simulink model "nigga"  (R2025a)
settings: Solver=VariableStepAuto  StartTime=0.0  StopTime=10.0  RelTol=1e-3
libraries: matlabinput_lib x1
settings Model: Creator=ASUS  LastModifiedBy=ASUS

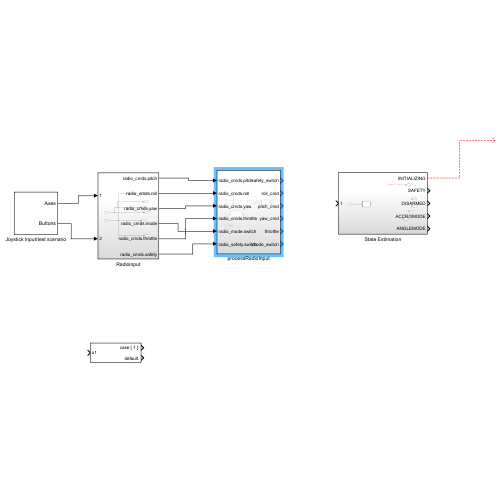
[thumbnail: Simulink's stored preview of the top-level diagram]
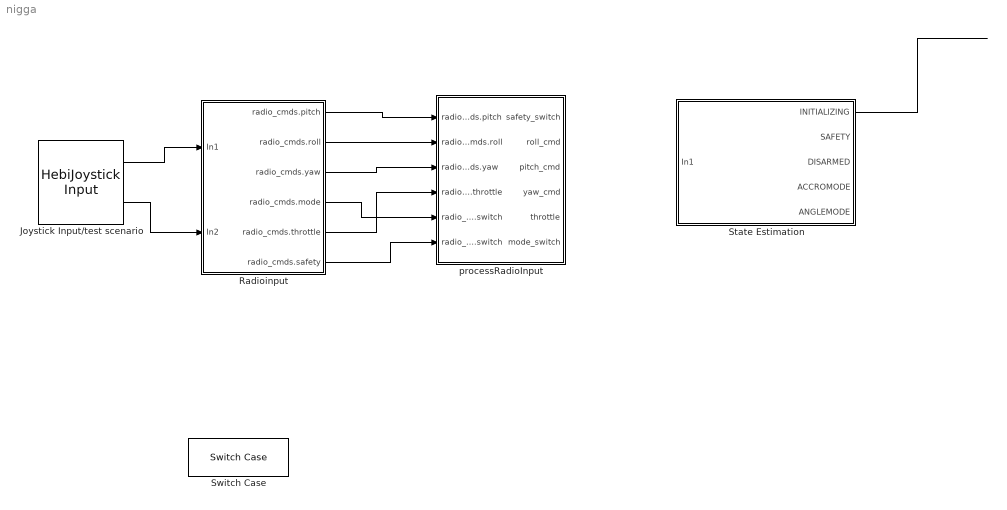
== system nigga ==
  Joystick Input/test scenario : matlabinput_lib/HebiJoystick Input  joyid=1  forcefeed=off
      settings: SourceProductName=MatlabInput
  Radioinput : Subsystem
  State Estimation : Subsystem
  Switch Case : SwitchCase
  processRadioInput : Subsystem
  wires:
  State Estimation/1(INITIALIZING) -> ?
  Joystick Input/test scenario/1 -> Radioinput/1(In1)
  Joystick Input/test scenario/2 -> Radioinput/2(In2)
  Radioinput/1(radio_cmds.pitch) -> processRadioInput/1(radio_cmds.pitch)
  Radioinput/2(radio_cmds.roll) -> processRadioInput/2(radio_cmds.roll)
  Radioinput/3(radio_cmds.yaw) -> processRadioInput/3(radio_cmds.yaw)
  Radioinput/5(radio_cmds.throttle) -> processRadioInput/4(radio_cmds.throttle)
  Radioinput/6(radio_cmds.safety) -> processRadioInput/6(radio_safety.switch)
  Radioinput/4(radio_cmds.mode) -> processRadioInput/5(radio_mode.switch)

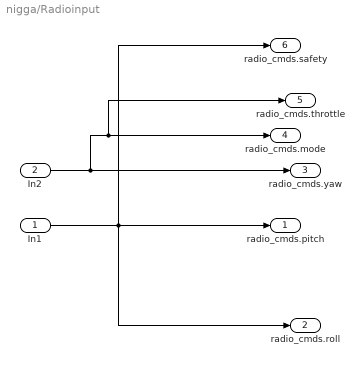
== system nigga/Radioinput ==
  In1 : Inport
  In2 : Inport  Port=2
  radio_cmds.pitch : Outport
  radio_cmds.roll : Outport  Port=2
  radio_cmds.yaw : Outport  Port=3
  radio_cmds.mode : Outport  Port=4
  radio_cmds.throttle : Outport  Port=5
  radio_cmds.safety : Outport  Port=6
  wires:
  In1/1 -> radio_cmds.roll/1, radio_cmds.safety/1, radio_cmds.pitch/1
  In2/1 -> radio_cmds.throttle/1, radio_cmds.mode/1, radio_cmds.yaw/1

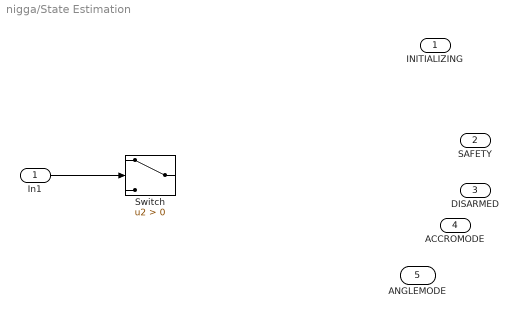
== system nigga/State Estimation ==
  In1 : Inport
  Switch : Switch  Criteria=u2 > Threshold  SaturateOnIntegerOverflow=off  InputSameDT=off
  INITIALIZING : Outport
  SAFETY : Outport  Port=2
  DISARMED : Outport  Port=3
  ACCROMODE : Outport  Port=4
  ANGLEMODE : Outport  Port=5
  wires:
  In1/1 -> Switch/2
  ? -> INITIALIZING/1

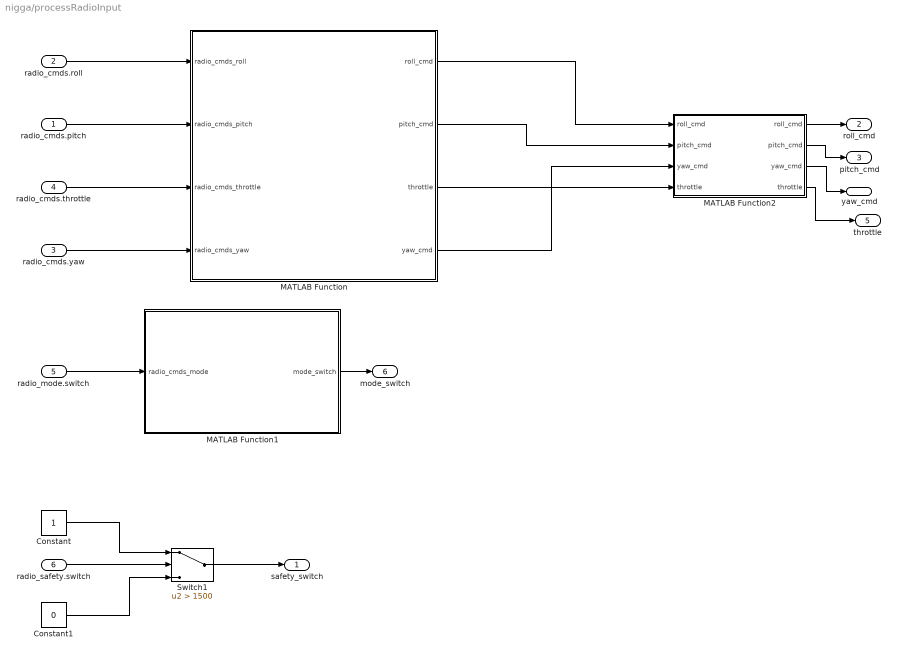
== system nigga/processRadioInput ==
  radio_cmds.pitch : Inport
  radio_cmds.roll : Inport  Port=2
  radio_cmds.yaw : Inport  Port=3
  radio_cmds.throttle : Inport  Port=4
  radio_mode.switch : Inport  Port=5
  radio_safety.switch : Inport  Port=6
  Constant : Constant
  Constant1 : Constant  Value=0
  MATLAB Function : MATLAB Function  TreatAsAtomicUnit=on
  MATLAB Function1 : MATLAB Function  TreatAsAtomicUnit=on
  MATLAB Function2 : MATLAB Function  TreatAsAtomicUnit=on
  Switch1 : Switch  Criteria=u2 > Threshold  Threshold=1500  SaturateOnIntegerOverflow=off  InputSameDT=off
  safety_switch : Outport
  roll_cmd : Outport  Port=2
  pitch_cmd : Outport  Port=3
  yaw_cmd : Outport  Port=4
  throttle : Outport  Port=5
  mode_switch : Outport  Port=6
  wires:
  radio_cmds.pitch/1 -> MATLAB Function/2(radio_cmds_pitch)
  radio_cmds.roll/1 -> MATLAB Function/1(radio_cmds_roll)
  radio_cmds.yaw/1 -> MATLAB Function/4(radio_cmds_yaw)
  radio_cmds.throttle/1 -> MATLAB Function/3(radio_cmds_throttle)
  MATLAB Function/1(roll_cmd) -> MATLAB Function2/1("roll_cmd ")
  MATLAB Function/2(pitch_cmd) -> MATLAB Function2/2("pitch_cmd ")
  MATLAB Function/3(throttle) -> MATLAB Function2/4("throttle ")
  MATLAB Function/4(yaw_cmd) -> MATLAB Function2/3("yaw_cmd ")
  MATLAB Function1/1(mode_switch) -> mode_switch/1
  radio_mode.switch/1 -> MATLAB Function1/1(radio_cmds_mode)
  radio_safety.switch/1 -> Switch1/2
  Constant1/1 -> Switch1/3
  Constant/1 -> Switch1/1
  Switch1/1 -> safety_switch/1
  MATLAB Function2/1(roll_cmd) -> roll_cmd/1
  MATLAB Function2/2(pitch_cmd) -> pitch_cmd/1
  MATLAB Function2/3(yaw_cmd) -> yaw_cmd/1
  MATLAB Function2/4(throttle) -> throttle/1

== matlab function nigga/processRadioInput/MATLAB Function1 ==
  data: radio_cmds_mode input; mode_switch output
function mode_switch = safetySwitch(radio_cmds_mode)


if radio_cmds_mode > 1700
       mode_switch = 1; % Angle mode
   elseif radio_cmds_mode < 1300
       mode_switch = 0; % Accro mode
   else
       mode_switch = 0; % Default to Accro

end

== matlab function nigga/processRadioInput/MATLAB Function ==
  data: radio_cmds_roll input; roll_cmd output; radio_cmds_pitch input; radio_cmds_throttle input; radio_cmds_yaw input; pitch_cmd output; throttle output; yaw_cmd output
function [roll_cmd, pitch_cmd, throttle, yaw_cmd]= scaleinputs(radio_cmds_roll,radio_cmds_pitch,radio_cmds_throttle,radio_cmds_yaw)
% Scale inputs to match your C++ code

   roll_cmd = (radio_cmds_roll - 1500) * 45 / 400;      % ±45 degrees
   pitch_cmd = (radio_cmds_pitch - 1500) * 45 / 400;    % ±45 degrees
   throttle = (radio_cmds_throttle - 1090) * 100 / 810; % 0-100%
   yaw_cmd = (radio_cmds_yaw - 1500) * 135 / 400;       % ±135 deg/s
end

== matlab function nigga/processRadioInput/MATLAB Function2 ==
  data: roll_cmd input; roll_cmd output; pitch_cmd output; yaw_cmd output; throttle output; pitch_cmd input; yaw_cmd input; throttle input
function [roll_cmd, pitch_cmd, yaw_cmd, throttle] = applyLimits(roll_cmd, pitch_cmd, yaw_cmd, throttle)

   roll_cmd = max(-45, min(45, roll_cmd));
   pitch_cmd = max(-45, min(45, pitch_cmd));
   yaw_cmd = max(-135, min(135, yaw_cmd));
   throttle = max(0, min(100, throttle));
end
